simulink library "RF"  (Simulink 4.00)
values from neighbouring files (symbols this model uses):
  A = rms(interp1(f,MX,fb))    [fftbandamp.m]    (also in logfft.m = fftamp(samples, fs, f, varargin{:})/vpp; plotfft.m = fftamp(samples, fs, f, varargin{:})*2/vpp)
  P = sinc((1575.42 - f)/10.23).^2./10.23    [L1PSD.m]    (also in fftphase.m = interp1(f,PX,f0))
undefined symbols (not defined in the file or in its folder): adb, B, CA_ID, fs, j, m, N, p, Phi, Range, Rice_K, Rice_Seed, Rice_Sigma, tau_delay, z
libraries: RF x133, dspcmplx x47, com_sour x8, dspelmat x8, com_chan x4, dspbdsp x3, dspswit x3, simulink_extras x2, com_filt x2
(part 1 of 5)
Description:
  | Blocks useful for simulation of wireless communication systems.  Originally intended for the simulation of
  | GPS transmitter, channel, and receiver, and later adapted for other uses.  This is a work in progress; no
  | claims or guarantees are made concerning accuracy, completeness, or fitness for any purpose.
settings Model: Creator=Jackson Harvey, Analog Design Group, University of Minnesota  LastModifiedBy=jharvey
settings Model: ModifiedComment=|
  | jharvey -- Mon Apr 16 18:15:06 2001 -- Version 1.15
  | Nonlinear transfer function was made compressive
settings Model: ModifiedHistory=|
  | jharvey -- Mon Apr 16 18:15:06 2001 -- Version 1.15
  | Nonlinear transfer function was made compressive
  | 
  | 
  | jharvey -- Fri Jan 19 15:13:26 2001 -- Version 1.14

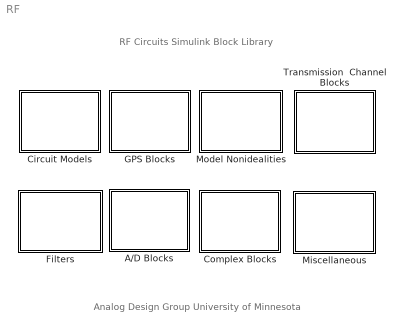
== system RF ==
  note: RF Circuits Simulink Block Library
  note: Analog Design Group
      | University of Minnesota
  A/D Blocks : Subsystem
      settings: RTWFcnNameOpts=Auto  RTWFileNameOpts=Auto
      mask Type: A/D Blocks
      mask Display: disp('A/D Blocks')
  Circuit Models : Subsystem
      settings: RTWFcnNameOpts=Auto  RTWFileNameOpts=Auto
      mask Type: RF Circuits
      mask Display: disp('RF Circuits')
  Complex Blocks : Subsystem
      settings: RTWFcnNameOpts=Auto  RTWFileNameOpts=Auto
      mask Type: Complex Blocks
      mask Display: disp('Complex Blocks')
  Filters : Subsystem
      settings: RTWFcnNameOpts=Auto  RTWFileNameOpts=Auto
      mask Type: Filters
      mask Display: disp('Filters')
  GPS Blocks : Subsystem
      settings: RTWFcnNameOpts=Auto  RTWFileNameOpts=Auto
      mask Type: GPS Blocks
      mask Display: disp('GPS Blocks')
  Miscellaneous : Subsystem
      settings: RTWFcnNameOpts=Auto  RTWFileNameOpts=Auto
      mask Type: Miscellaneous
      mask Display: disp('Miscellaneous')
  Model Nonidealities : Subsystem
      settings: RTWFcnNameOpts=Auto  RTWFileNameOpts=Auto
      mask Type: Nonidealities
      mask Display: disp('Nonidealities')
  Transmission  Channel Blocks : Subsystem
      settings: RTWFcnNameOpts=Auto  RTWFileNameOpts=Auto
      mask Type: Channel Blocks
      mask Display: disp('Channel Blocks')

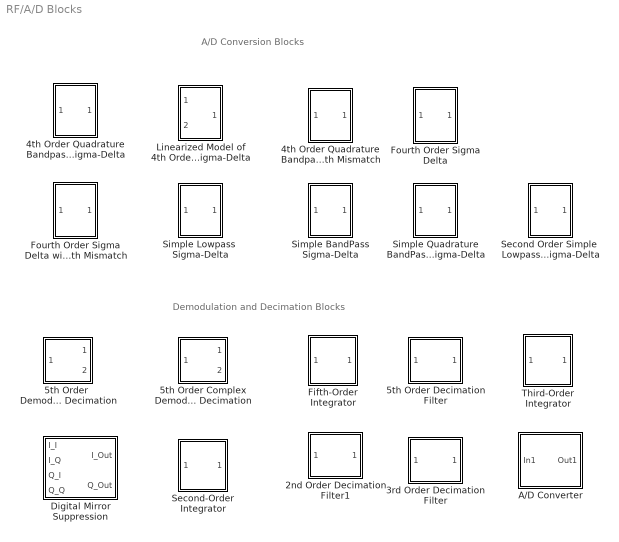
== system RF/A/D Blocks ==
  note: A/D Conversion Blocks
  note: Demodulation and Decimation Blocks
  2nd Order Decimation Filter1 : Subsystem  mask(Second Order Decimation Filter){N=32, fs=1E6}
      mask prompts: N "Decimation Factor (N)"; fs "Sampling Rate"
      mask help: Second Order Decimation Filter. Input is passed through asecond order 'integrate and dump' filter, and then downsampled.
      settings: RTWFcnNameOpts=Auto  RTWFileNameOpts=Auto
      mask Help: Second Order Decimation Filter.  Input is passed through asecond order 'integrate and dump' filter, and then downsampled.
      mask Display: plot(0,0,100,100,[10,20,20],[30,10,90],[30,20],[30,10],[80,80,40,40],[90,10,90,10])
  3rd Order Decimation Filter : Subsystem  mask(Third Order Decimation Filter){N=12, fs=1350E6*2}
      mask prompts: N "Decimation Factor (N)"; fs "Sampling Rate"
      mask help: Third Order Decimation Filter. Input is passed through a third order 'integrate and dump' filter, and then downsampled.
      settings: RTWFcnNameOpts=Auto  RTWFileNameOpts=Auto
      mask Help: Second Order Decimation Filter.  Input is passed through a thirdd order 'integrate and dump' filter, and then downsampled.
      mask Display: plot(0,0,100,100,[10,20,20],[30,10,90],[30,20],[30,10],[80,80,40,40],[90,10,90,10])
  4th Order Quadrature Bandpass Sigma-Delta : Subsystem  mask(Fourth Order Quadrature Bandpass Sigma-Delta){NTF_Poles=conj([0.67605+0.28003i 0.84752+0.10317i 0.67224+0.52633i 0.87023-0.35538i]), NTF_Zeros=conj([0.94544+0.3258i 0.92388+0.38268i 0.8989+0.43815i 0.92388-0.38268i]), STF_Zeros=conj([0.79335-0.60876i 0.13053+0.99144i 0.87023-0.35538i]), STF_Gain=0.95, fs=80E6}
      mask prompts: NTF_Poles "Noise Transfer Function Poles (4)"; NTF_Zeros "Noise Transfer Function Zeros (4)"; STF_Zeros "Signal Transfer Function Zeros (3)"; STF_Gain "Maximum Signal Gain (usually 1)"; fs "Sampling Frequency"
      mask help: Fourth Order Quadrature Bandpass Sigma-Delta. After Stephen Jantzi, "Quadrature Bandpass Delta-Sigma Modulation for Digital Radio," Ph.D. dissertation, University of Toronto. More information on parameters can be found in the above reference.
      mask init:
      | ts = 1/fs;
      | 
      | [H,W]=freqz(poly(STF_Zeros),poly(NTF_Poles));
      | k = -STF_Gain / max(H);
      | 
      | % Calculate modulator coefficients
      | d = real(NTF_Zeros) - 1;
      | c = imag(NTF_Zeros);
      | 
      | Beta = poly(NTF_Poles);
      | z = NTF_Zeros;
      | B(4) = - (z(4)+z(3)+z(2)+z(1)) - Beta(2);
      | B(3)=B(4)*(z(3)+z(2)+z(1))+z(4)*z(3)+z(4)*z(2)+z(4)*z(1)+z(3)*z(2);
      | B(3) = B(3)+z(3)*z(1)+z(2)*z(1)-Beta(3);
      | B(2) = -B(4)*(z(3)*z(2)+z(3)*z(1)+z(2)*z(1)) + B(3)*(z(2)+z(1));
      | B(2) = B(2) - (z(4)*z(3)*z(2)+z(4)*z(3)*z(1)+z(4)*z(2)*z(1)+z(3)*z(2)*z(1)) - Beta(4);
      | B(1) = B(4)*z(3)*z(2)*z(1) - B(3)*z(2)*z(1) + B(2)*z(1);
      | B(1) = B(1) + z(4)*z(3)*z(2)*z(1) - Beta(5);
      | b = real(B);
      | f = imag(B);
      | 
      | Alpha = k*poly(STF_Zeros);
      | A(4) = Alpha(1);
      | A(3) = A(4)*(z(3)+z(2)+z(1)) + Alpha(2);
      | A(2) = -A(4)*(z(3)*z(2)+z(3)*z(1)+z(2)*z(1)) + A(3)*(z(2)+z(1)) + Alpha(3);
      | A(1) = A(4)*z(3)*z(2)*z(1) - A(3)*z(2)*z(1) + A(2)*z(1) + Alpha(4);
      | a = real(A);
      | e = imag(A);
      settings: RTWFcnNameOpts=Auto  RTWFileNameOpts=Auto
      mask Help: Fourth Order Quadrature Bandpass Sigma-Delta.  After Stephen Jantzi, "Quadrature Bandpass Delta-Sigma Modulation for Digital Radio," Ph.D. dissertation, University of Toronto.  More information on parameters can be found in the above reference.
      mask Display: plot(0,0,100,100,[40,10],[80,80],[40,10,20,10,40],[40,40,60,80,80],[50,90,70,50],[40,40,80,40])
  4th Order Quadrature Bandpass Sigma-Delta with Mismatch : Subsystem  mask(Fourth Order Quadrature Bandpass Sigma-Delta with Mismatch){NTF_Poles=conj([0.67605+0.28003i 0.84752+0.10317i 0.67224+0.52633i 0.87023-0.35538i]), NTF_Zeros=conj([0.94544+0.3258i 0.92388+0.38268i 0.8989+0.43815i 0.92388-0.38268i]), STF_Zeros=conj([0.79335-0.60876i 0.13053+0.99144i 0.87023-0.35538i]), STF_Gain=0.95, ErrorStd=1, fs=80E6}
      mask prompts: NTF_Poles "Noise Transfer Function Poles (4)"; NTF_Zeros "Noise Transfer Function Zeros (4)"; STF_Zeros "Signal Transfer Function Zeros (3)"; STF_Gain "Maximum Signal Gain (usually 1)"; ErrorStd "Coefficient Standard Error (Percent Nominal Value)"; fs "Sampling Frequency"
      mask help: Fourth Order Quadrature Bandpass Sigma-Delta. After Stephen Jantzi, "Quadrature Bandpass Delta-Sigma Modulation for Digital Radio," Ph.D. dissertation, University of Toronto. More information on parameters can be found in the above reference.
      mask init:
      | ts = 1/fs;
      | 
      | [H,W]=freqz(poly(STF_Zeros),poly(NTF_Poles));
      | k = -STF_Gain / max(H);
      | 
      | % Calculate modulator coefficients
      | d = real(NTF_Zeros) - 1;
      | c = imag(NTF_Zeros);
      | 
      | Beta = poly(NTF_Poles);
      | z = NTF_Zeros;
      | B(4) = - (z(4)+z(3)+z(2)+z(1)) - Beta(2);
      | B(3)=B(4)*(z(3)+z(2)+z(1))+z(4)*z(3)+z(4)*z(2)+z(4)*z(1)+z(3)*z(2);
      | B(3) = B(3)+z(3)*z(1)+z(2)*z(1)-Beta(3);
      | B(2) = -B(4)*(z(3)*z(2)+z(3)*z(1)+z(2)*z(1)) + B(3)*(z(2)+z(1));
      | B(2) = B(2) - (z(4)*z(3)*z(2)+z(4)*z(3)*z(1)+z(4)*z(2)*z(1)+z(3)*z(2)*z(1)) - Beta(4);
      | B(1) = B(4)*z(3)*z(2)*z(1) - B(3)*z(2)*z(1) + B(2)*z(1);
      | B(1) = B(1) + z(4)*z(3)*z(2)*z(1) - Beta(5);
      | b = real(B);
      | f = imag(B);
      | 
      | Alpha = k*poly(STF_Zeros);
      | A(4) = Alpha(1);
      | A(3) = A(4)*(z(3)+z(2)+z(1)) + Alpha(2);
      | A(2) = -A(4)*(z(3)*z(2)+z(3)*z(1)+z(2)*z(1)) + A(3)*(z(2)+z(1)) + Alpha(3);
      | A(1) = A(4)*z(3)*z(2)*z(1) - A(3)*z(2)*z(1) + A(2)*z(1) + Alpha(4);
      | a = real(A);
      | e = imag(A);
      | 
      | a = a + a .* ErrorStd/100 .* randn(1, length(a));
      | b = b + b .* ErrorStd/100 .* randn(1,length(b));
      | c1 = c + c .* ErrorStd/100 .* randn(1,length(c));
      | c2 = c + c .* ErrorStd/100 .* randn(1,length(c));
      | d1 = d + d .* ErrorStd/100 .* randn(1,length(d));
      | d2 = d + d .* ErrorStd/100 .* randn(1,length(d));
      | e = e + e .* ErrorStd/100 .* randn(1,length(e));
      | f = f + f .* ErrorStd/100 .* randn(1,length(f));
      settings: RTWFcnNameOpts=Auto  RTWFileNameOpts=Auto
      mask Help: Fourth Order Quadrature Bandpass Sigma-Delta.  After Stephen Jantzi, "Quadrature Bandpass Delta-Sigma Modulation for Digital Radio," Ph.D. dissertation, University of Toronto.  More information on parameters can be found in the above reference.
      mask Display: plot(0,0,100,100,[40,10],[80,80],[40,10,20,10,40],[40,40,60,80,80],[50,90,70,50],[40,40,80,40])
  5th Order Decimation Filter : Subsystem  mask(Fifth Order Decimation Filter){N=32, fs=1E6}
      mask prompts: N "Decimation Factor (N)"; fs "Sampling Rate"
      mask help: Fifth Order Decimation Filter. Input is passed through a fifth order 'integrate and dump' filter, and then downsampled.
      settings: RTWFcnNameOpts=Auto  RTWFileNameOpts=Auto
      mask Help: Fifth Order Decimation Filter.  Input is passed through a fifth order 'integrate and dump' filter, and then downsampled.
      mask Display: plot(0,0,100,100,[10,20,20],[30,10,90],[30,20],[30,10],[80,80,40,40],[90,10,90,10])
  5th Order  Demodulation and Decimation : Subsystem  mask(Decimation And Demodulation){fs=10E6, fIF=3.75E6, N=25}
      mask prompts: fs "Sampling Frequency"; fIF "IF Frequency"; N "Decimation Factor (N)"
      mask help: Demodulates the output of a bandpass sigma delta and decimates by a factor N. Each channel (I and Q) is decimated by a factor 2N. The result is a baseband complex signal sampled at 1/N the input sampling frequency.
      settings: RTWFcnNameOpts=Auto  RTWFileNameOpts=Auto
      mask Help: Demodulates the output of a bandpass sigma delta and decimates by a factor N.  Each channel (I and Q) is decimated by a factor 2N.  The result is a baseband complex signal sampled at 1/N the input sampling frequency.
      mask Display:
      | plot(0,0,100,100,[24,20,15,20,20],[85,95,85,95,20],[80,20,95,85,95,85],[70,20,20,15,20,24],[56,56,55,52,50,46],[20,26,31,35,38,42]);
      | text(95,85,'I'); text(95,30,'Q');
  5th Order Complex Demodulation and Decimation : Subsystem  mask(Complex Decimation And Demodulation){fs=10E6, fIF=3.75E6, N=25}
      mask prompts: fs "Sampling Frequency"; fIF "IF Frequency"; N "Decimation Factor (N)"
      mask help: Demodulates the output of a quadrature bandpass sigma delta and decimates by a factor N. Each channel (I and Q) is decimated by a factor 2N. The result is a baseband complex signal sampled at 1/N the input sampling frequency.
      settings: RTWFcnNameOpts=Auto  RTWFileNameOpts=Auto
      mask Help: Demodulates the output of a quadrature bandpass sigma delta and decimates by a factor N.  Each channel (I and Q) is decimated by a factor 2N.  The result is a baseband complex signal sampled at 1/N the input sampling frequency.
      mask Display:
      | plot(0,0,100,100,[24,20,15,20,20],[85,95,85,95,20],[80,20,95,85,95,85],[70,20,20,15,20,24],[56,56,55,52,50,46],[20,26,31,35,38,42]);
      | text(95,85,'I'); text(95,30,'Q');
  A/D Converter : Subsystem  mask(Ideal A/D Converter){FSlevel=1, signed=off, fs=2048, N=2, el=on}
      mask prompts: FSlevel "Full-Scale Output Range"; signed "Signed Input?"; fs "Sampling Frequency"; N "Number of Bits"; el "Extra Level?"
      mask help: Performs A/D Conversion. Full-scale output range is full-scale input range - 1 LSB. In other words, 1 LSB is full-scale input range / 2^N, which is full-scale output range / 2^N - 1. The zero level is midtread for unsigned input.
      mask init:
      | N = round(N);
      | qlevel = FSlevel/(2^N-1 + el);
      | ilevel = signed*FSlevel/2;
      | slevel = (2^N - 1 + el)/FSlevel;
      settings: RTWFcnNameOpts=Auto  RTWFileNameOpts=Auto
      mask Help: Performs A/D Conversion.  Full-scale output range is full-scale input range - 1 LSB.  In other words, 1 LSB is full-scale input range / 2^N, which is full-scale output range / 2^N - 1.  The zero level is midtread for unsigned input.
      mask Display: disp('Ideal A/D')
  Digital Mirror Suppression : Subsystem  mask(Digital Image Suppression){S=Signal Higher than LO}
      mask prompts: S "Mask Parameter 1:"
      mask help: Perform Image Suppression in the digital domain for the low IF receiver topology. The inputs are the I and Q signals of both the I and Q branches. For instance, 'I,Q' is the Q output of the I channel.
      mask init:
      | if (S==1),
      |   g1=1; g2=-1;
      | end;
      | if (S==2),
      |   g1=-1;g2=1;
      | end;
      settings: RTWFcnNameOpts=Auto  RTWFileNameOpts=Auto
      mask Help: Perform Image Suppression in the digital domain for the low IF receiver topology.  The inputs are the I and Q signals of both the I and Q branches. For instance, 'I,Q' is the Q output of the I channel.
      mask StyleString: popup(Signal Higher than LO|Signal Lower than LO)
      mask Display:
      | plot(0,0,100,100,[50,50,90,10],[90,50,50,50],[70,70],[60,50],[80,75,65,60],[50,80,80,49]); text(5,35,'Q,I'); text(5,7,'Q,Q')
      | text(95,15,'Q'); text(98,80,'I'); text(5,95,'I,I'), text(5, 70,'I,Q');
  Fifth-Order Integrator : Subsystem  mask(Fifth Order Integrate and Dump){fs=10E6, N=25}
      mask prompts: fs "Sampling Frequency"; N "Decimation Ratio (N)"
      mask help: Fifth Order Integrate and Dump Filter.
      settings: RTWFcnNameOpts=Auto  RTWFileNameOpts=Auto
      mask Help: Fifth Order Integrate and Dump Filter.
      mask Display: plot(0,0,100,100,[60,70,20,40,20,70,60],[70,90,90,50,10,10,30])
  Fourth Order Sigma Delta : Subsystem  mask(Fourth Order Sigma-Delta){NTF_Poles=[0.73497-0.20683i 0.73497+0.20683i 0.73442-0.47052i 0.73442+0.47052i], NTF_Zeros=[0.94028-0.34041i 0.94028+0.34041i 0.90558-0.42417i 0.90558+0.42417i], STF_Zeros=[inf inf inf], STF_Gain=0.85, fs=64E6}
      mask prompts: NTF_Poles "NTF Poles (4 poles)"; NTF_Zeros "NTF Zeros (4 zeros)"; STF_Zeros "STF Zeros (3 Zeros)"; STF_Gain "Max STF Gain (usually 1)"; fs "Sampling Frequency"
      mask help: Fourth Order Sigma Delta Modulator utilizing the 'cascade of resonators with distributed feedback' architecture. For poles or zeros at infinity enter inf. Proper poles and zeros can be calculated using R. Shreier's Delta-Sigma Toolbox.
      mask init:
      | ts = 1/fs;
      | if (abs(1-cumprod(NTF_Zeros)) > 0.05),
      |   error('Invalid Noise Transfer Zeros');
      | end;
      | 
      | if (length(NTF_Zeros) ~= 4),
      |   error('Invalid Noise Transfer Zeros');
      | end;
      | 
      | if (length(NTF_Poles) ~= 4),
      |   error('Invalid Noise Transfer Poles');
      | end;
      | 
      | if (length(STF_Zeros) ~= 3),
      |   error('Invalid Signal Transfer Poles');
      | end;
      | 
      | NTFZ = cplxpair(NTF_Zeros);
      | temp = poly([NTFZ(1) NTFZ(2)]);
      | c(1) = temp(2) + 2;
      | temp = poly([NTFZ(3) NTFZ(4)]);
      | c(2) = temp(2) + 2;
      | 
      | k = STF_Gain / max(abs(freqz(poly(STF_Zeros), poly(NTF_Poles))));
      | STF_Num = [zeros(1,4-length(poly(STF_Zeros))) k*poly(STF_Zeros)];
      | 
      | a(4) =  - STF_Num(4);
      | a(3) = STF_Num(1) - a(4);
      | a(2) = -1 * (STF_Num(3) - a(3) - 3*a(4) + c(1)*a(4));
      | a(1) = STF_Num(2) - a(2) + 3*a(4) - c(1)*a(4) - c(1)*a(3) + 2*a(3);
      | 
      | NTF_Denom = [zeros(1,5-length(poly(NTF_Poles))) poly(NTF_Poles)];
      | 
      | b(4) = 1 - NTF_Denom(5);
      | b(3) = NTF_Denom(2) - b(4) - c(1) - c(2) + 4;
      | b(2) = -1 * (NTF_Denom(4) - c(1) - b(3) + 4 - c(2) + c(1)*b(4) - 3*b(4));
      | b(1) = NTF_Denom(3) + 2*c(1) + 3*b(4) + 2*c(2) + 2*b(3) - b(2) - c(1)*c(2) - c(1)*b(4) - c(1)*b(3) - 6;
      | 
      | A = real(a);
      | B = real(b);
      | G = real(c);
      settings: RTWFcnNameOpts=Auto  RTWFileNameOpts=Auto
      mask Help: Fourth Order Sigma Delta Modulator utilizing the 'cascade of resonators with distributed feedback' architecture..  For poles or zeros at infinity enter inf.  Proper poles and zeros can be calculated using R. Shreier's Delta-Sigma Toolbox.
      mask Display: plot(0,0,100,100,[40,10],[80,80],[40,10,20,10,40],[40,40,60,80,80],[50,90,70,50],[40,40,80,40])
  Fourth Order Sigma Delta with Mismatch : Subsystem  mask(Fourth Order Sigma-Delta){NTF_Poles=[0.73497-0.20683i 0.73497+0.20683i 0.73442-0.47052i 0.73442+0.47052i], NTF_Zeros=[0.94028-0.34041i 0.94028+0.34041i 0.90558-0.42417i 0.90558+0.42417i], STF_Zeros=[inf inf inf], STF_Gain=0.85, ErrorStd=1, fs=64E6}
      mask prompts: NTF_Poles "NTF Poles (4 poles)"; NTF_Zeros "NTF Zeros (4 zeros)"; STF_Zeros "STF Zeros (3 Zeros)"; STF_Gain "Max STF Gain (usually 1)"; ErrorStd "Coefficient Error Standard Deviation (Percent Nominal Value)"; fs "Sampling Frequency"
      mask help: Fourth Order Sigma Delta Modulator utilizing the 'cascade of resonators with distributed feedback' architecture. For poles or zeros at infinity enter inf. Proper poles and zeros can be calculated using R. Shreier's Delta-Sigma Toolbox. Gaussian coefficient error with mean zero and variable standard deviation is added to simulate capacitor variation.
      mask init:
      | ts = 1/fs;
      | if (abs(1-cumprod(NTF_Zeros)) > 0.05),
      |   error('Invalid Noise Transfer Zeros');
      | end;
      | 
      | if (length(NTF_Zeros) ~= 4),
      |   error('Invalid Noise Transfer Zeros');
      | end;
      | 
      | if (length(NTF_Poles) ~= 4),
      |   error('Invalid Noise Transfer Poles');
      | end;
      | 
      | if (length(STF_Zeros) ~= 3),
      |   error('Invalid Signal Transfer Poles');
      | end;
      | 
      | NTFZ = cplxpair(NTF_Zeros);
      | temp = poly([NTFZ(1) NTFZ(2)]);
      | c(1) = temp(2) + 2;
      | temp = poly([NTFZ(3) NTFZ(4)]);
      | c(2) = temp(2) + 2;
      | 
      | k = STF_Gain / max(abs(freqz(poly(STF_Zeros), poly(NTF_Poles))));
      | STF_Num = [zeros(1,4-length(poly(STF_Zeros))) k*poly(STF_Zeros)];
      | 
      | a(4) =  - STF_Num(4);
      | a(3) = STF_Num(1) - a(4);
      | a(2) = -1 * (STF_Num(3) - a(3) - 3*a(4) + c(1)*a(4));
      | a(1) = STF_Num(2) - a(2) + 3*a(4) - c(1)*a(4) - c(1)*a(3) + 2*a(3);
      | 
      | NTF_Denom = [zeros(1,5-length(poly(NTF_Poles))) poly(NTF_Poles)];
      | 
      | b(4) = 1 - NTF_Denom(5);
      | b(3) = NTF_Denom(2) - b(4) - c(1) - c(2) + 4;
      | b(2) = -1 * (NTF_Denom(4) - c(1) - b(3) + 4 - c(2) + c(1)*b(4) - 3*b(4));
      | b(1) = NTF_Denom(3) + 2*c(1) + 3*b(4) + 2*c(2) + 2*b(3) - b(2) - c(1)*c(2) - c(1)*b(4) - c(1)*b(3) - 6;
      | 
      | A = real(a);
      | B = real(b);
      | G = real(c);
      | 
      | A = A + A .* (ErrorStd/100) .* randn(1,length(A));
      | B = B + B .* (ErrorStd/100) .* randn(1,length(B));
      | G = G + G .* (ErrorStd/100) .* randn(1,length(G));
      settings: RTWFcnNameOpts=Auto  RTWFileNameOpts=Auto
      mask Help: Fourth Order Sigma Delta Modulator utilizing the 'cascade of resonators with distributed feedback' architecture..  For poles or zeros at infinity enter inf.  Proper poles and zeros can be calculated using R. Shreier's Delta-Sigma Toolbox.  Gaussian coefficient error with mean zero and variable standard deviation is added to simulate capacitor variation.
      mask Display: plot(0,0,100,100,[40,10],[80,80],[40,10,20,10,40],[40,40,60,80,80],[50,90,70,50],[40,40,80,40])
  Linearized Model of 4th Order Quadrature Bandpass Sigma-Delta : Subsystem  mask(Linear Model of Fourth Order Quadrature Bandpass Sigma-Delta){NTF_Zeros=conj([0.67605+0.28003i 0.84752+0.10317i 0.67224+0.52633i 0.87023-0.35538i]), NTF_Poles=conj([0.94544+0.3258i 0.92388+0.38268i 0.8989+0.43815i 0.92388-0.38268i]), STF_Zeros=conj([0.79335-0.60876i 0.13053+0.99144i 0.87023-0.35538i]), STF_Gain=0.95, ErrorStd=1, Seed=7, fs=80E6}
      mask prompts: NTF_Zeros "Noise Transfer Function Zeros (4)"; NTF_Poles "Noise Transfer Function Poles (4)"; STF_Zeros "Signal Transfer Function Zeros (3)"; STF_Gain "Maximum Signal Gain (usually 1)"; ErrorStd "Coefficient Standard Deviation (Percent Nominal Value)"; Seed "Error Seed"; fs "Sampling Frequency"
      mask help: Linear model of Fourth Order Quadrature Bandpass Sigma-Delta. After Stephen Jantzi, "Quadrature Bandpass Delta-Sigma Modulation for Digital Radio," Ph.D. dissertation, University of Toronto. Used for finding the transfer functions of modulator when mismatch is considered. More information on parameters can be found in the above reference.
      mask init:
      | ts = 1/fs;
      | 
      | [H,W]=freqz(poly(STF_Zeros),poly(NTF_Poles));
      | k = -STF_Gain / max(H);
      | 
      | % Calculate modulator coefficients
      | d = real(NTF_Zeros) - 1;
      | c = imag(NTF_Zeros);
      | 
      | Beta = poly(NTF_Poles);
      | z = NTF_Zeros;
      | B(4) = - (z(4)+z(3)+z(2)+z(1)) - Beta(2);
      | B(3)=B(4)*(z(3)+z(2)+z(1))+z(4)*z(3)+z(4)*z(2)+z(4)*z(1)+z(3)*z(2);
      | B(3) = B(3)+z(3)*z(1)+z(2)*z(1)-Beta(3);
      | B(2) = -B(4)*(z(3)*z(2)+z(3)*z(1)+z(2)*z(1)) + B(3)*(z(2)+z(1));
      | B(2) = B(2) - (z(4)*z(3)*z(2)+z(4)*z(3)*z(1)+z(4)*z(2)*z(1)+z(3)*z(2)*z(1)) - Beta(4);
      | B(1) = B(4)*z(3)*z(2)*z(1) - B(3)*z(2)*z(1) + B(2)*z(1);
      | B(1) = B(1) + z(4)*z(3)*z(2)*z(1) - Beta(5);
      | b = real(B);
      | f = imag(B);
      | 
      | Alpha = k*poly(STF_Zeros);
      | A(4) = Alpha(1);
      | A(3) = A(4)*(z(3)+z(2)+z(1)) + Alpha(2);
      | A(2) = -A(4)*(z(3)*z(2)+z(3)*z(1)+z(2)*z(1)) + A(3)*(z(2)+z(1)) + Alpha(3);
      | A(1) = A(4)*z(3)*z(2)*z(1) - A(3)*z(2)*z(1) + A(2)*z(1) + Alpha(4);
      | a = real(A);
      | e = imag(A);
      | 
      | randn('seed', Seed);
      | a = a + a .* ErrorStd/100 .* randn(1, length(a));
      | b = b + b .* ErrorStd/100 .* randn(1,length(b));
      | c1 = c + c .* ErrorStd/100 .* randn(1,length(c));
      | c2 = c + c .* ErrorStd/100 .* randn(1,length(c));
      | d1 = d + d .* ErrorStd/100 .* randn(1,length(d));
      | d2 = d + d .* ErrorStd/100 .* randn(1,length(d));
      | e = e + e .* ErrorStd/100 .* randn(1,length(e));
      | f = f + f .* ErrorStd/100 .* randn(1,length(f));
      settings: RTWFcnNameOpts=Auto  RTWFileNameOpts=Auto
      mask Help: Linear model of Fourth Order Quadrature Bandpass Sigma-Delta.  After Stephen Jantzi, "Quadrature Bandpass Delta-Sigma Modulation for Digital Radio," Ph.D. dissertation, University of Toronto.  Used for finding the transfer functions of modulator when mismatch is considered.  More information on parameters can be found in the above reference.
      mask Display: plot(0,0,100,100,[40,10],[80,80],[40,10,20,10,40],[40,40,60,80,80],[50,90,70,50],[40,40,80,40])
  Second Order Simple  Lowpass  Sigma-Delta : Subsystem  mask(Second Order Lowpass Sigma Delta){fs=1E6}
      mask prompts: fs "Sampling Frequency"
      mask help: Second Order Lowpass Sigma Delta Modulator with noise pole at 0.
      settings: RTWFcnNameOpts=Auto  RTWFileNameOpts=Auto
      mask Help: Second Order Lowpass Sigma Delta Modulator with noise pole at 0.
      mask Display: plot(0,0,100,100,[40,10],[80,80],[40,10,20,10,40],[40,40,60,80,80],[50,90,70,50],[40,40,80,40])
  Second-Order Integrator : Subsystem  mask(Second Order Integrate and Dump){fs=fs, N=N}
      mask prompts: fs "Sampling Frequency"; N "Decimation Ratio (N)"
      mask help: Second Order Integrate and Dump Filter.
      settings: RTWFcnNameOpts=Auto  RTWFileNameOpts=Auto
      mask Help: Second Order Integrate and Dump Filter.
      mask Display: plot(0,0,100,100,[60,70,20,40,20,70,60],[70,90,90,50,10,10,30])
  Simple BandPass Sigma-Delta : Subsystem  mask(Simple Bandpass Sigma Delta){fs=1E6}
      mask prompts: fs "Sampling Frequency"
      mask help: Bandpass Sigma Delta with noise poles at fs/4.
      settings: RTWFcnNameOpts=Auto  RTWFileNameOpts=Auto
      mask Help: Bandpass Sigma Delta with noise poles at fs/4.
      mask Display: plot(0,0,100,100,[40,10],[80,80],[40,10,20,10,40],[40,40,60,80,80],[50,90,70,50],[40,40,80,40])
  Simple Lowpass  Sigma-Delta : Subsystem  mask(First Order Lowpass Sigma Delta){fs=1E6}
      mask prompts: fs "Sampling Frequency"
      mask help: First Order Lowpass Sigma Delta Modulator with noise pole at 0.
      settings: RTWFcnNameOpts=Auto  RTWFileNameOpts=Auto
      mask Help: First Order Lowpass Sigma Delta Modulator with noise pole at 0.
      mask Display: plot(0,0,100,100,[40,10],[80,80],[40,10,20,10,40],[40,40,60,80,80],[50,90,70,50],[40,40,80,40])
  Simple Quadrature BandPass Sigma-Delta : Subsystem  mask(Quadrature Bandpass Sigma Delta){fs=1E6}
      mask prompts: fs "Sampling Frequency"
      mask help: Quadrature Bandpass Sigma Delta.
      mask init:
      | ts = 1/fs;
      settings: RTWFcnNameOpts=Auto  RTWFileNameOpts=Auto
      mask Help: Quadrature Bandpass Sigma Delta.
      mask Display: plot(0,0,100,100,[40,10],[80,80],[40,10,20,10,40],[40,40,60,80,80],[50,90,70,50],[40,40,80,40])
  Third-Order Integrator : Subsystem  mask(Third Order Integrate and Dump){fs=fs, N=N}
      mask prompts: fs "Sampling Frequency"; N "Decimation Ratio (N)"
      mask help: Third Order Integrate and Dump Filter.
      settings: RTWFcnNameOpts=Auto  RTWFileNameOpts=Auto
      mask Help: Third Order Integrate and Dump Filter.
      mask Display: plot(0,0,100,100,[60,70,20,40,20,70,60],[70,90,90,50,10,10,30])

== system RF/Circuit Models ==
  note: RF Circuit Models
  Clock  with Jitter : Subsystem  mask(Clock with Jitter){f0=99.99, DCycle=0.5, Phase0=0, PError=1, Seed=1, VHigh=1, VLow=-1}
      mask prompts: f0 "Frequency (Hz)"; DCycle "Duty Cycle"; Phase0 "Initial Phase (rad)"; PError "Peak Percent Jitter"; Seed "Jitter Seed"; VHigh "Output High"; VLow "Output Low"
      mask help: Clock with a variable frequency, output level, duty cycle, and initial phase. Jitter which is Gaussian in time is added which has "peak" jitter in time as a percentage of clock period.
      settings: RTWFcnNameOpts=Auto  RTWFileNameOpts=Auto
      mask Help: Clock with a variable frequency, output level, duty cycle, and initial phase.  Jitter which is Gaussian in time is added which has "peak" jitter in time as a percentage of clock period.
      mask Display: plot(0,0,100,100,[95,90,90,75,75,60,60,45,45,30,30,15,15,5],[25,25,75,75,25,25,75,75,25,25,75,75,25,25]);
  Clock  without Jitter : Subsystem  mask(Clock Without Jitter){f0=99.99, DCycle=0.5, Phase0=0, VHigh=1, VLow=-1, PError=1}
      mask prompts: f0 "Frequency (Hz)"; DCycle "Duty Cycle"; Phase0 "Initial Phase (rad)"; VHigh "Output High"; VLow "Output Low"; PError "Peak % Error of Jittered Clock"
      mask help: Clock with a variable frequency, output level, duty cycle, and initial phase. Used as a metric for the clock with jitter, as well as for an ideal clock.
      settings: RTWFcnNameOpts=Auto  RTWFileNameOpts=Auto
      mask Help: Clock with a variable frequency, output level, duty cycle, and initial phase.  Used as a metric for the clock with jitter, as well as for an ideal clock.
      mask Display: plot(0,0,100,100,[95,90,90,75,75,60,60,45,45,30,30,15,15,5],[25,25,75,75,25,25,75,75,25,25,75,75,25,25]);
  Comparator : Subsystem  mask(Comparator){L_Out=-1, H_Out=1, Bound=0}
      mask prompts: L_Out "Low Output"; H_Out "High Output"; Bound "Boundary"
      mask help: Outputs "low" level when the input is less than the boundary setting, and "high" when the input is above the boundary setting.
      settings: RTWFcnNameOpts=Auto  RTWFileNameOpts=Auto
      mask Help: Outputs "low" level when the input is less than the boundary setting, and "high" when the input is above the boundary setting.
      mask Display: plot(0,0,100,100,[50,50],[0,100],[100,0],[50,50],[100,50],[80,80],[50,-0],[20,20])
  Comparator with Hysteresis : Subsystem  mask(Comparator with Hysteresis){L_Out=-1, H_Out=1, Bound=0, NPeak=0.25}
      mask prompts: L_Out "Low Output"; H_Out "High Output"; Bound "Boundary"; NPeak "Peak Noise"
      mask help: Comparator
      settings: RTWFcnNameOpts=Auto  RTWFileNameOpts=Auto
      mask Help: Outputs "low" level when the input is less than the boundary setting, and "high" when the input is above the boundary setting.
      mask Display: plot(0,0,100,100,[50,50],[0,100],[100,0],[50,50],[30,30,100,70,70,0],[20,80,80,80,20,20],[75,70,65],[65,70,65],[25,30,35],[35,30,35])
  Non-Ideal Mixer : Subsystem  mask(Mixer with Nonidealities){Gain1=0, IIP2=-500, IIP3=-500, fmax=1200, V1dB=1.5, AWGNVRMS=1E-12, SeedAWGN=1, Fseed=2, f0=1000, N0=1.147E-7, fm=10E3, numtaps=100}
      mask prompts: Gain1 "Primary Gain (dBV)"; IIP2 "Second Order Intercept (dBV)"; IIP3 "Third Order Intercept (dBV)"; fmax "Max. Output Frequency (Hz)"; V1dB "1 dB Compression Voltage (dBV)"; AWGNVRMS "Output Referred Noise VRMS"; SeedAWGN "White Noise Seed"; Fseed "Flicker Noise Seed"; f0 "Flicker Noise Reference Frequency (Hz)"; N0 "Flicker Noise Reference Voltage (V/Hz^0.5)"; fm "Maximum Flicker Noise Frequency (Hz)"; numtaps "Number of Taps for Flicker Noise"
      mask help: Mixer with nonidealities. Small signal nonlinearity, compression, saturation, slew rate limiting, and noise (white and flicker) are modeled. For more information about each nonideality, see the documentation of the nonlinear transfer function block, the compression block, and the flicker noise block, and that of the built-in blocks: saturation, rate limiting, and additive white gaussian noise.
      settings: RTWFcnNameOpts=Auto  RTWFileNameOpts=Auto
      mask Help: Mixer with nonidealities.  Small signal nonlinearity, compression, saturation, slew rate limiting, and noise (white and flicker) are modeled.  For more information about each nonideality, see the documentation of the nonlinear transfer function block, the compression block, and the flicker noise block, and that of the built-in blocks: saturation, rate limiting, and additive white gaussian noise.
      mask Display: plot(0,0,100,100,[90,10],[90,10],[90,10],[10,90])
  Non-Ideal  LNA : Subsystem  mask(LNA){Gain1=0, IIP2=30, IIP3=20, AWGNVRMS=1E-3, fmax=3E9, V1dB=-4, SeedAWGN=123, FSeed=2, f0=1000, N0=1.147E-7, fm=10E3, numtaps=100}
      mask prompts: Gain1 "Primary Gain (dB)"; IIP2 "Second Order Intercept (dB)"; IIP3 "Third Order Intercept (dB)"; AWGNVRMS "Output Referred Noise VRMS"; fmax "Maximum Frequency"; V1dB "1 dB Compression Voltage (dB)"; SeedAWGN "Noise Seed"; FSeed "Flicker Noise Seed"; f0 "Flicker Noise Reference Frequency (Hz)"; N0 "Flicker Noise Reference Amplitude (V/Hz^0.5)"; fm "Maximum Flicker Noise Frequency (Hz)"; numtaps "Number of Taps for Flicker Noise"
      mask help: Low Noise Amplifier with nonidealities. Small signal nonlinearity, compression, saturation, slew rate limiting, and noise (white and flicker) are modeled. For more information about each nonideality, see the documentation of the nonlinear transfer function block, the compression block, and the flicker noise block, and that of the built-in blocks: saturation, rate limiting, and additive white gaussian noise.
      settings: RTWFcnNameOpts=Auto  RTWFileNameOpts=Auto
      mask Help: Low Noise Amplifier with nonidealities.  Small signal nonlinearity, compression, saturation, slew rate limiting, and noise (white and flicker) are modeled.  For more information about each nonideality, see the documentation of the nonlinear transfer function block, the compression block, and the flicker noise block, and that of the built-in blocks: saturation, rate limiting, and additive white gaussian noise.
      mask Display:
      | plot(0,0,100,100,[0,100,0,0],[100,50,0,100])
      | disp('LNA')
  Quadrature Oscillator : Subsystem  mask(Quadrature Oscillator){PhiE=deg2rad(2), AE=adb(0.1), Phi=0, A=1, f0=1575.42E6}
      mask prompts: PhiE "Phase Error (radians)"; AE "Amplitude Error"; Phi "Common Phase (radians)"; A "Common Amplitude"; f0 "Frequency (Hz)"
      mask help: Quadrature Oscillator with fixed amplitude and phase error between signals. The I signal and the Q signal are offset by 90 degrees - phase error. The I amplitude is (1 + amplitude error) as large as the Q signal. A shared phase can be set to simulate noncoherent systems.
      settings: RTWFcnNameOpts=Auto  RTWFileNameOpts=Auto
      mask Help: Quadrature Oscillator with fixed amplitude and phase error between signals.  The I signal and the Q signal are offset by 90 degrees - phase error.  The I amplitude is (1 + amplitude error) as large as the Q signal.  A shared phase can be set to simulate noncoherent systems.
      mask Display:
      | plot([-1:1/8:1]*0.75,sin(0:pi/8:2*pi),[-0.5:1/8:1.5]*0.75,sin(0:pi/8:2*pi)*0.75);
      | text(1.1,0.6,'I');text(1,-0.6,'Q');
  Simple Non-Ideal Mixer : Subsystem  mask(Mixer with Nonidealities){Gain1=0, IIP2=-500, IIP3=-500, AWGNVRMS=1E-12, SeedAWGN=1}
      mask prompts: Gain1 "Primary Gain (dBV)"; IIP2 "Second Order Intercept (dBV)"; IIP3 "Third Order Intercept (dBV)"; AWGNVRMS "Output Referred Noise VRMS"; SeedAWGN "White Noise Seed"
      mask help: Mixer with nonidealities. Small signal nonlinearity, compression, saturation, slew rate limiting, and noise (white and flicker) are modeled. For more information about each nonideality, see the documentation of the nonlinear transfer function block, the compression block, and the flicker noise block, and that of the built-in blocks: saturation, rate limiting, and additive white gaussian noise.
      settings: RTWFcnNameOpts=Auto  RTWFileNameOpts=Auto
      mask Help: Mixer with nonidealities.  Small signal nonlinearity, compression, saturation, slew rate limiting, and noise (white and flicker) are modeled.  For more information about each nonideality, see the documentation of the nonlinear transfer function block, the compression block, and the flicker noise block, and that of the built-in blocks: saturation, rate limiting, and additive white gaussian noise.
      mask Display: plot(0,0,100,100,[90,10],[90,10],[90,10],[10,90])
  Simple Non-Ideal  LNA : Subsystem  mask(LNA){Gain1=0, IIP2=30, IIP3=20, AWGNVRMS=1E-3, SeedAWGN=123}
      mask prompts: Gain1 "Primary Gain (dB)"; IIP2 "Second Order Intercept (dB)"; IIP3 "Third Order Intercept (dB)"; AWGNVRMS "Output Referred Noise VRMS"; SeedAWGN "Noise Seed"
      mask help: Low Noise Amplifier with nonidealities. Small signal nonlinearity, compression, saturation, slew rate limiting, and noise (white and flicker) are modeled. For more information about each nonideality, see the documentation of the nonlinear transfer function block, the compression block, and the flicker noise block, and that of the built-in blocks: saturation, rate limiting, and additive white gaussian noise.
      settings: RTWFcnNameOpts=Auto  RTWFileNameOpts=Auto
      mask Help: Low Noise Amplifier with nonidealities.  Small signal nonlinearity, compression, saturation, slew rate limiting, and noise (white and flicker) are modeled.  For more information about each nonideality, see the documentation of the nonlinear transfer function block, the compression block, and the flicker noise block, and that of the built-in blocks: saturation, rate limiting, and additive white gaussian noise.
      mask Display:
      | plot(0,0,100,100,[0,100,0,0],[100,50,0,100])
      | disp('LNA')

== system RF/Complex Blocks ==
  note: Complex Blocks
  Complex Gain : Subsystem  mask(Complex Gain){G=1+j}
      mask prompts: G "Gain"
      mask help: Multiply a complex input by a complex constant.
      settings: RTWFcnNameOpts=Auto  RTWFileNameOpts=Auto
      mask Help: Multiply a complex input by a complex constant.
      mask Display: disp(G);
  Complex Quantizer : Subsystem  mask(Complex Comparator){L_Out_C=-1, H_Out_C=1, Bound_C=0}
      mask prompts: L_Out_C "Low Output"; H_Out_C "High Output"; Bound_C "Boundary"
      mask help:
      | Switch between two output levels based on the input level.  Each
      | component of the complex signal is independently quantized and then
      | the components are recombined to form the output.
      settings: RTWFcnNameOpts=Auto  RTWFileNameOpts=Auto
      mask Help:
      | Switch between two output levels based on the input level.  Each
      | component of the complex signal is independently quantized and then
      | the components are recombined to form the output.
      mask Display: plot(0,0,100,100,[50,50],[0,100],[100,0],[50,50],[100,50],[70,70],[50,-0],[30,30])
  Complex Unit Delay : Subsystem  mask(Complex Unit Delay){icr=1, ici=1, ts=0.001}
      mask prompts: icr "Real Initial Output"; ici "Imaginary Initial Output"; ts "Sample Time"
      mask help: Delays a complex input by one sample period.
      settings: RTWFcnNameOpts=Auto  RTWFileNameOpts=Auto
      mask Help: Delays a complex input by one sample period.
      mask Display: disp('1/z')
  Complex  Continuous Pole : Subsystem  mask(Continuous Time Complex Pole){d=1, c=1}
      mask help: Continuous Time Complex Pole. Implements the transfer function 1/(s-d-j*c)
      settings: RTWFcnNameOpts=Auto  RTWFileNameOpts=Auto
      mask Help: Continuous Time Complex Pole.   Implements the transfer function 1/(s-d-j*c)
      mask Display: disp('Complex \nContinuous \nPole')
  "Complex Continuous Pole with Mismatch " : Subsystem  mask(Continuous Time Complex Pole with Mismatch){c1=0.99, c2=1.05, d1=0.97, d2=1.01}
      mask help: Continuous Time Complex Pole. Implements the transfer function 1/(s-d-j*c). Mismatch between coefficients is modelled by perturbing c and d to form c1,c2 and d1,d2.
      settings: RTWFcnNameOpts=Auto  RTWFileNameOpts=Auto
      mask Help: Continuous Time Complex Pole.   Implements the transfer function 1/(s-d-j*c).  Mismatch between coefficients is modelled by perturbing c and d to form c1,c2 and d1,d2.
      mask Display: disp('Complex \nContinuous \nPole')
  Complex Pole : Subsystem  mask(Complex Pole){c=0.5, d=0.5, ts=0.001}
      mask prompts: ts "Sample Time"
      mask help: Implements the transfer function 1/(z - (1+d+jc)) on a complex input to give a complex output. After Stephen Jantzi, "Quadrature Bandpass Delta-Sigma Modulation for Digital Radio," Ph.D. Dissertation, University of Toronto.
      settings: RTWFcnNameOpts=Auto  RTWFileNameOpts=Auto
      mask Help: Implements the transfer function 1/(z - (1+d+jc)) on a complex input to give a complex output.  After Stephen Jantzi, "Quadrature Bandpass Delta-Sigma Modulation for Digital Radio," Ph.D. Dissertation, University of Toronto.
      mask Display: disp('Complex\n Discrete Pole')
  Complex Pole with Mismatch : Subsystem  mask(Complex Pole with Mismatch){c1=0.43, c2=0.55, d1=0.42, d2=0.53, ts=0.001}
      mask prompts: ts "Sample Time"
      mask help: Implements the transfer function 1/(z - (1+d+jc)) on a complex input to give a complex output. After Stephen Jantzi, "Quadrature Bandpass Delta-Sigma Modulation for Digital Radio," Ph.D. Dissertation, University of Toronto. Mismatch is implemented using slightly perturbed values for each copy of parameters.
      settings: RTWFcnNameOpts=Auto  RTWFileNameOpts=Auto
      mask Help: Implements the transfer function 1/(z - (1+d+jc)) on a complex input to give a complex output.  After Stephen Jantzi, "Quadrature Bandpass Delta-Sigma Modulation for Digital Radio," Ph.D. Dissertation, University of Toronto.  Mismatch is implemented using slightly perturbed values for each copy of parameters.
      mask Display: disp('Complex\n Discrete Pole\nwith Mismatch')
  Complex Random  Number : Subsystem  mask(Complex Random Number){Mean=0, Sigma=1, Seeds=[5 7]}
      mask prompts: Seeds "Seeds (two integers)"
      mask help: Complex Random Number
      settings: RTWFcnNameOpts=Auto  RTWFileNameOpts=Auto
      mask Help: Complex Random Number
      mask Display: plot( rand(1,31)*20);
